simulink model "moteurs"  (R2025b)
settings: Solver=VariableStepAuto  StartTime=0.0  StopTime=200  RelTol=1e-3
values from neighbouring files (symbols this model uses):
  alpha = 10    [variables.m]
  J = 10    [variables.m]
  Ke = 200    [variables.m]
  Kth = 800    [variables.m]
  n_IDL = 600    [variables.m]
  tau_ACY = (2*n_IDL*C/T)*(2*pi/60)    (= 251.327412287)    [variables.m]
  tau_e = 0.01    [variables.m]
  tau_th = 0.4    [variables.m]
  Td_th = 0.02    [variables.m]
settings Model: Creator=flo  LastModifiedBy=flo

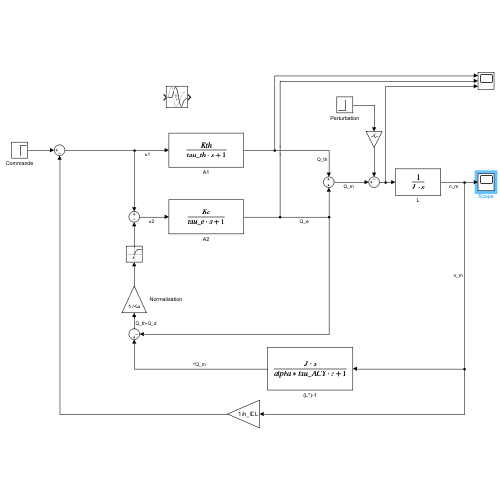
[thumbnail: Simulink's stored preview of the top-level diagram]
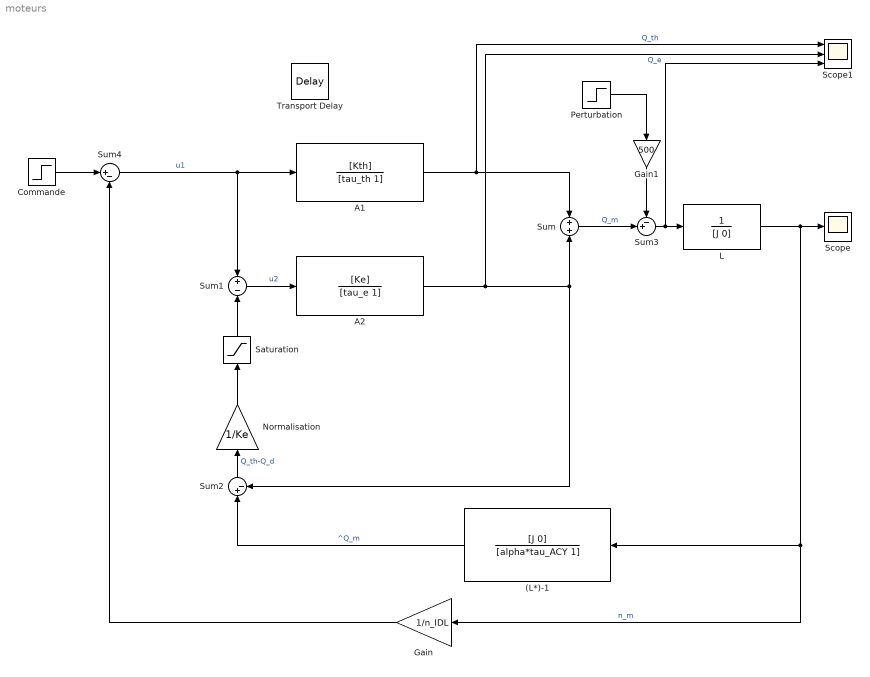
== system moteurs ==
  (L*)-1 : TransferFcn  Numerator=[J 0]  Denominator=[alpha*tau_ACY 1]
  A1 : TransferFcn  Numerator=[Kth]  Denominator=[tau_th 1]
  A2 : TransferFcn  Numerator=[Ke]  Denominator=[tau_e 1]
  Commande : Step  Time=0  SampleTime=0
  Gain : Gain  Gain=1/n_IDL
  Gain1 : Gain  Gain=500
  L : TransferFcn  Denominator=[J 0]
  Normalisation : Gain  Gain=1/Ke
  Perturbation : Step  Time=100  SampleTime=0
  Saturation : Saturate  UpperLimit=1  LowerLimit=0
  Scope : Scope
      settings: ActiveDisplayYMinimum=-74.196228987404623  ActiveDisplayYMaximum=667.76606088664175
  Scope1 : Scope  NumInputPorts=3
      settings: ActiveDisplayYMinimum=-671.1140733861339  ActiveDisplayYMaximum=1031.8884756095561
  Sum : Sum  Inputs=+|+
  Sum1 : Sum  Inputs=+|-
  Sum2 : Sum  Inputs=|+-
  Sum3 : Sum  Inputs=-+|
  Sum4 : Sum  Inputs=|+-
  Transport Delay : TransportDelay  DelayTime=Td_th
  wires:
  A1/1 -> Scope1/1, Sum/1  "Q_th"
  Sum4/1 -> Sum1/1, A1/1  "u1"
  Sum1/1 -> A2/1  "u2"
  Sum2/1 -> Normalisation/1  "Q_th-Q_d"
  Sum/1 -> Sum3/2  "Q_m"
  Perturbation/1 -> Gain1/1
  Sum3/1 -> Scope1/3, L/1
  L/1 -> (L*)-1/1, Gain/1, Scope/1  "n_m"
  Commande/1 -> Sum4/1
  Gain/1 -> Sum4/2
  A2/1 -> Scope1/2, Sum2/2, Sum/2  "Q_e"
  (L*)-1/1 -> Sum2/1  "^Q_m"
  Normalisation/1 -> Saturation/1
  Gain1/1 -> Sum3/1
  Saturation/1 -> Sum1/2
